simulink model "RotorParams"  (R2020b)
settings: Solver=VariableStepAuto  StartTime=0.0  StopTime=600  RelTol=1e-3
undefined symbols (not defined in the file): rho, Vehicle
libraries: simulink x1, dynamicsLibrary x1
settings Model: Creator=dbell44  LastModifiedBy=dbell44

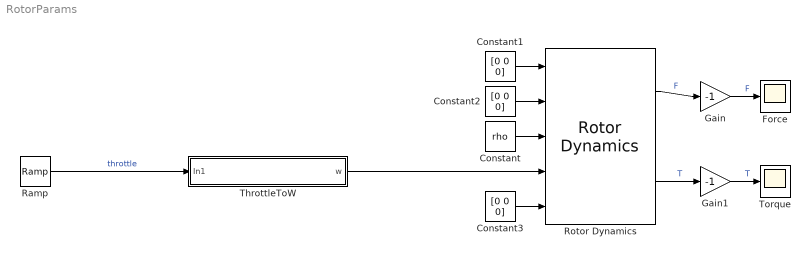
== system RotorParams ==
  Constant : Constant  Value=rho  VectorParams1D=off
  Constant1 : Constant  Value=[0 0 0]
  Constant2 : Constant  Value=[0 0 0]
  Constant3 : Constant  Value=[0 0 0]
  Force : Scope
  Gain : Gain  Gain=-1
  Gain1 : Gain  Gain=-1
  Ramp : simulink/Sources/Ramp  slope=1  start=0  InitialOutput=0
  Rotor Dynamics : dynamicsLibrary/Rotor Dynamics  SystemSampleTime=-1  VariantActivationTime=update diagram  Latency=0  AutoFrameSizeCalculation=off
  ThrottleToW : Subsystem
  Torque : Scope
  wires:
  Ramp/1 -> ThrottleToW/1(In1)  "throttle"
  ThrottleToW/1(w) -> Rotor Dynamics/4
  Constant/1 -> Rotor Dynamics/3
  Constant2/1 -> Rotor Dynamics/2
  Constant1/1 -> Rotor Dynamics/1
  Constant3/1 -> Rotor Dynamics/5
  Rotor Dynamics/1 -> Gain/1  "F"
  Rotor Dynamics/2 -> Gain1/1  "T"
  Gain1/1 -> Torque/1  "T"
  Gain/1 -> Force/1  "F"

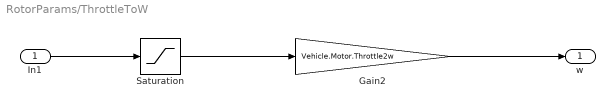
== system RotorParams/ThrottleToW ==
  In1 : Inport
  Gain2 : Gain  Gain=Vehicle.Motor.Throttle2w
  Saturation : Saturate  UpperLimit=Vehicle.Motor.maxSignal  LowerLimit=Vehicle.Motor.minSignal  LinearizeAsGain=off
  w : Outport
  wires:
  In1/1 -> Saturation/1
  Saturation/1 -> Gain2/1
  Gain2/1 -> w/1
